simulink library "SIXOSEM_T_STAGE_MASTER"  (Simulink 8.0)
settings: Solver=ode45  StartTime=0.0  StopTime=10.0  RelTol=1e-3
libraries: cdsEpicsOut x51, cdsFilt x31, cdsTP x24, cdsFiltCtrl x9, cdsEpicsIn x9, cdsMuxMatrix x5, cdsEpicsBinIn x2, SIXOSEM_T_COILOUTF_MASTER x1, cdsFunctionCall x1, SIXOSEM_T_WD_AC_MASTER x1
(part 1 of 5)
settings Model: Creator=controls  LastModifiedBy=stuart.aston

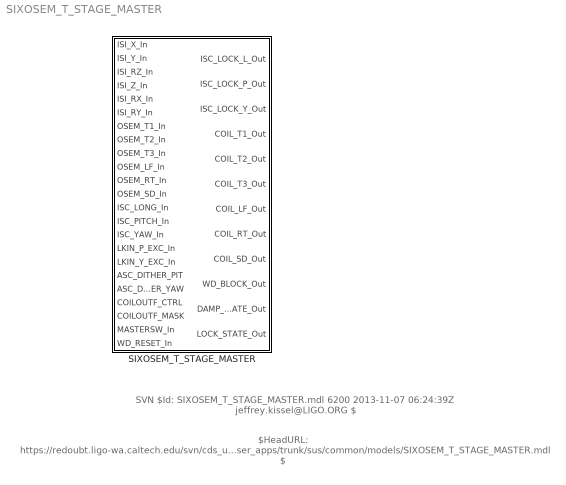
== system SIXOSEM_T_STAGE_MASTER ==
  note: $HeadURL: https://redoubt.ligo-wa.caltech.edu/svn/cds_user_apps/trunk/sus/common/models/SIXOSEM_T_STAGE_MASTER.mdl $
  note: SVN $Id: SIXOSEM_T_STAGE_MASTER.mdl 6200 2013-11-07 06:24:39Z jeffrey.kissel@LIGO.ORG $
  SIXOSEM_T_STAGE_MASTER : Subsystem  Description=SIXOSEMSTAGE_FACE_MASTER

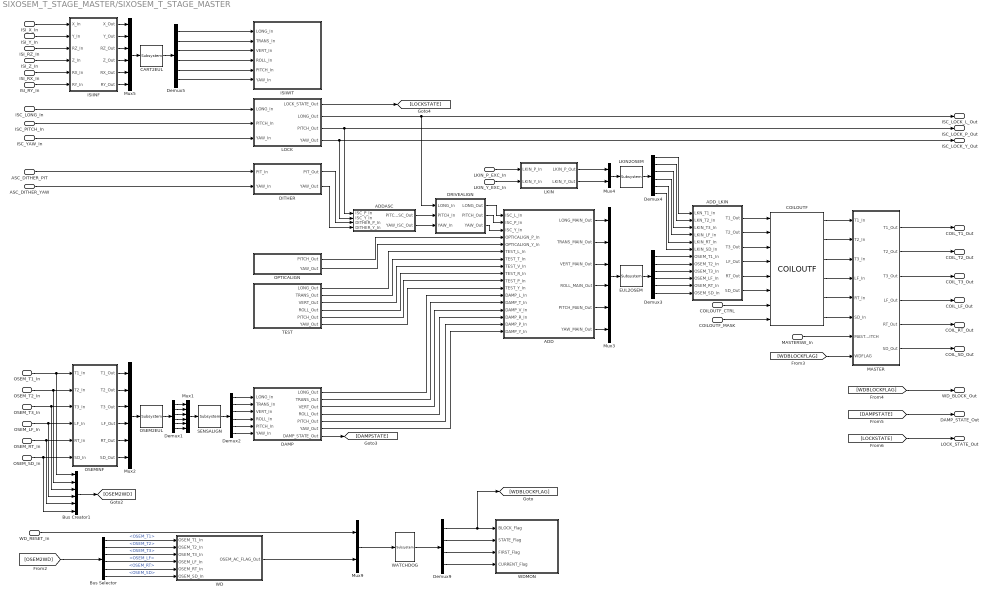
== system SIXOSEM_T_STAGE_MASTER/SIXOSEM_T_STAGE_MASTER ==
  ISI_X_In : Inport
  ISI_Y_In : Inport  Port=2
  ISI_RZ_In : Inport  Port=3
  ISI_Z_In : Inport  Port=4
  ISI_RX_In : Inport  Port=5
  ISI_RY_In : Inport  Port=6
  OSEM_T1_In : Inport  Port=7
  OSEM_T2_In : Inport  Port=8
  OSEM_T3_In : Inport  Port=9
  OSEM_LF_In : Inport  Port=10
  OSEM_RT_In : Inport  Port=11
  OSEM_SD_In : Inport  Port=12
  ISC_LONG_In : Inport  Port=13
  ISC_PITCH_In : Inport  Port=14
  ISC_YAW_In : Inport  Port=15
  LKIN_P_EXC_In : Inport  Port=16
  LKIN_Y_EXC_In : Inport  Port=17
  ASC_DITHER_PIT : Inport  Port=18
  ASC_DITHER_YAW : Inport  Port=19
  COILOUTF_CTRL : Inport  Port=20
  COILOUTF_MASK : Inport  Port=21
  MASTERSW_In : Inport  Port=22
  WD_RESET_In : Inport  Port=23
  ADD : Subsystem
  ADDASC : Subsystem
  ADD_LKIN : Subsystem
  Bus Creator1 : BusCreator  Inputs='OSEM_T1','OSEM_T2','OSEM_T3','OSEM_LF','OSEM_RT','OSEM_SD'
  Bus Selector : BusSelector  OutputSignals=OSEM_T1,OSEM_T2,OSEM_T3,OSEM_LF,OSEM_RT,OSEM_SD
  CART2EUL : cdsMuxMatrix/Subsystem  Tag=cdsMuxMatrix  Description=Any size matrix. Inputs and outputs must be connected using Mux and Demux parts.
      settings: AttributesFormatString=%<Tag>
  COILOUTF : SIXOSEM_T_COILOUTF_MASTER/COILOUTF
  DAMP : Subsystem
  DITHER : Subsystem
  DRIVEALIGN : Subsystem
  Demux{1..5} (5 alike) : Demux  Outputs=6
  Demux9 : Demux
  EUL2OSEM : cdsMuxMatrix/Subsystem  Tag=cdsMuxMatrix  Description=Any size matrix. Inputs and outputs must be connected using Mux and Demux parts.
      settings: AttributesFormatString=%<Tag>
  ISIINF : Subsystem
  ISIWIT : Subsystem
  LKIN : Subsystem
  LKIN2OSEM : cdsMuxMatrix/Subsystem  Tag=cdsMuxMatrix  Description=Any size matrix. Inputs and outputs must be connected using Mux and Demux parts.
      settings: AttributesFormatString=%<Tag>
  LOCK : Subsystem
  MASTER : Subsystem
  Mux{1..3,5} (4 alike) : Mux  Inputs=6
  Mux4 : Mux  Inputs=2
  Mux9 : Mux  Inputs=2
  OPTICALIGN : Subsystem
  OSEM2EUL : cdsMuxMatrix/Subsystem  Tag=cdsMuxMatrix  Description=Any size matrix. Inputs and outputs must be connected using Mux and Demux parts.
      settings: AttributesFormatString=%<Tag>
  OSEMINF : Subsystem
  SENSALIGN : cdsMuxMatrix/Subsystem  Tag=cdsMuxMatrix  Description=Any size matrix. Inputs and outputs must be connected using Mux and Demux parts.
      settings: AttributesFormatString=%<Tag>
  TEST : Subsystem
  WATCHDOG : cdsFunctionCall/Subsystem  Tag=cdsFunctionCall  Description=inline OSEMWATCHDOG $SUS_SRC/WATCHDOG.c
      settings: AttributesFormatString=%<Tag>\n%<Description>
  WD : Subsystem
  WDMON : Subsystem
  ISC_LOCK_L_Out : Outport
  ISC_LOCK_P_Out : Outport  Port=2
  ISC_LOCK_Y_Out : Outport  Port=3
  COIL_T1_Out : Outport  Port=4
  COIL_T2_Out : Outport  Port=5
  COIL_T3_Out : Outport  Port=6
  COIL_LF_Out : Outport  Port=7
  COIL_RT_Out : Outport  Port=8
  COIL_SD_Out : Outport  Port=9
  WD_BLOCK_Out : Outport  Port=10
  DAMP_STATE_Out : Outport  Port=11
  LOCK_STATE_Out : Outport  Port=12
  wires:
  WATCHDOG/1 -> Demux9/1
  Mux9/1 -> WATCHDOG/1
  COILOUTF/6 -> MASTER/6(SD_In)
  COILOUTF/5 -> MASTER/5(RT_In)
  COILOUTF/4 -> MASTER/4(LF_In)
  COILOUTF/3 -> MASTER/3(T3_In)
  COILOUTF/2 -> MASTER/2(T2_In)
  COILOUTF/1 -> MASTER/1(T1_In)
  Demux9/4 -> WDMON/4(CURRENT_Flag)
  Demux9/3 -> WDMON/3(FIRST_Flag)
  Demux9/2 -> WDMON/2(STATE_Flag)
  Demux9/1 -> [WDBLOCKFLAG], WDMON/1(BLOCK_Flag)
  EUL2OSEM/1 -> Demux3/1
  Mux3/1 -> EUL2OSEM/1
  MASTER/6(SD_Out) -> COIL_SD_Out/1
  MASTER/5(RT_Out) -> COIL_RT_Out/1
  MASTER/4(LF_Out) -> COIL_LF_Out/1
  MASTER/3(T3_Out) -> COIL_T3_Out/1
  MASTER/2(T2_Out) -> COIL_T2_Out/1
  MASTER/1(T1_Out) -> COIL_T1_Out/1
  SENSALIGN/1 -> Demux2/1
  Mux1/1 -> SENSALIGN/1
  Demux1/6 -> Mux1/6
  Demux1/5 -> Mux1/5
  Demux1/4 -> Mux1/4
  Demux1/3 -> Mux1/3
  Demux1/2 -> Mux1/2
  Demux1/1 -> Mux1/1
  OSEM2EUL/1 -> Demux1/1
  Bus Selector/6 -> WD/6(OSEM_SD_In)  "<OSEM_SD>"
  Bus Selector/5 -> WD/5(OSEM_RT_In)  "<OSEM_RT>"
  Bus Selector/4 -> WD/4(OSEM_LF_In)  "<OSEM_LF>"
  Bus Selector/3 -> WD/3(OSEM_T3_In)  "<OSEM_T3>"
  Bus Selector/2 -> WD/2(OSEM_T2_In)  "<OSEM_T2>"
  Bus Selector/1 -> WD/1(OSEM_T1_In)  "<OSEM_T1>"
  [OSEM2WD] -> Bus Selector/1
  Bus Creator1/1 -> [OSEM2WD]
  ISC_YAW_In/1 -> LOCK/3(YAW_In)
  ISC_PITCH_In/1 -> LOCK/2(PITCH_In)
  ISC_LONG_In/1 -> LOCK/1(LONG_In)
  Mux2/1 -> OSEM2EUL/1
  OSEM_SD_In/1 -> Bus Creator1/6, OSEMINF/6(SD_In)
  OSEM_RT_In/1 -> Bus Creator1/5, OSEMINF/5(RT_In)
  OSEM_LF_In/1 -> Bus Creator1/4, OSEMINF/4(LF_In)
  OSEM_T3_In/1 -> Bus Creator1/3, OSEMINF/3(T3_In)
  OSEM_T2_In/1 -> Bus Creator1/2, OSEMINF/2(T2_In)
  OSEM_T1_In/1 -> Bus Creator1/1, OSEMINF/1(T1_In)
  OSEMINF/1(T1_Out) -> Mux2/1
  OSEMINF/2(T2_Out) -> Mux2/2
  OSEMINF/3(T3_Out) -> Mux2/3
  OSEMINF/4(LF_Out) -> Mux2/4
  OSEMINF/5(RT_Out) -> Mux2/5
  OSEMINF/6(SD_Out) -> Mux2/6
  ISI_X_In/1 -> ISIINF/1(X_In)
  ISI_Y_In/1 -> ISIINF/2(Y_In)
  ISI_RZ_In/1 -> ISIINF/3(RZ_In)
  ISI_Z_In/1 -> ISIINF/4(Z_In)
  ISI_RX_In/1 -> ISIINF/5(RX_In)
  ISI_RY_In/1 -> ISIINF/6(RY_In)
  ISIINF/1(X_Out) -> Mux5/1
  ISIINF/2(Y_Out) -> Mux5/2
  ISIINF/3(RZ_Out) -> Mux5/3
  ISIINF/4(Z_Out) -> Mux5/4
  ISIINF/5(RX_Out) -> Mux5/5
  ISIINF/6(RY_Out) -> Mux5/6
  Mux5/1 -> CART2EUL/1
  CART2EUL/1 -> Demux5/1
  Demux5/1 -> ISIWIT/1(LONG_In)
  Demux5/2 -> ISIWIT/2(TRANS_In)
  Demux5/3 -> ISIWIT/3(VERT_In)
  Demux5/4 -> ISIWIT/4(ROLL_In)
  Demux5/5 -> ISIWIT/5(PITCH_In)
  Demux5/6 -> ISIWIT/6(YAW_In)
  [WDBLOCKFLAG] -> MASTER/8(WDFLAG)
  Demux2/1 -> DAMP/1(LONG_In)
  Demux2/2 -> DAMP/2(TRANS_In)
  Demux2/3 -> DAMP/3(VERT_In)
  Demux2/4 -> DAMP/4(ROLL_In)
  Demux2/5 -> DAMP/5(PITCH_In)
  Demux2/6 -> DAMP/6(YAW_In)
  [WDBLOCKFLAG] -> WD_BLOCK_Out/1
  DAMP/7(DAMP_STATE_Out) -> [DAMPSTATE]
  [DAMPSTATE] -> DAMP_STATE_Out/1
  ADD/1(LONG_MAIN_Out) -> Mux3/1
  ADD/2(TRANS_MAIN_Out) -> Mux3/2
  ADD/3(VERT_MAIN_Out) -> Mux3/3
  ADD/4(ROLL_MAIN_Out) -> Mux3/4
  ADD/5(PITCH_MAIN_Out) -> Mux3/5
  ADD/6(YAW_MAIN_Out) -> Mux3/6
  LOCK/1(LOCK_STATE_Out) -> [LOCKSTATE]
  [LOCKSTATE] -> LOCK_STATE_Out/1
  LKIN/1(LKIN_P_Out) -> Mux4/1
  LKIN2OSEM/1 -> Demux4/1
  Mux4/1 -> LKIN2OSEM/1
  ADD_LKIN/1(T1_Out) -> COILOUTF/1
  ADD_LKIN/2(T2_Out) -> COILOUTF/2
  ADD_LKIN/3(T3_Out) -> COILOUTF/3
  ADD_LKIN/4(LF_Out) -> COILOUTF/4
  ADD_LKIN/5(RT_Out) -> COILOUTF/5
  ADD_LKIN/6(SD_Out) -> COILOUTF/6
  Demux4/1 -> ADD_LKIN/1(LKN_T1_In)
  Demux4/2 -> ADD_LKIN/2(LKN_T2_In)
  Demux4/3 -> ADD_LKIN/3(LKIN_T3_In)
  Demux4/4 -> ADD_LKIN/4(LKIN_LF_In)
  Demux4/5 -> ADD_LKIN/5(LKIN_RT_In)
  Demux4/6 -> ADD_LKIN/6(LKIN_SD_In)
  Demux3/1 -> ADD_LKIN/7(OSEM_T1_In)
  Demux3/2 -> ADD_LKIN/8(OSEM_T2_In)
  Demux3/3 -> ADD_LKIN/9(OSEM_T3_In)
  Demux3/4 -> ADD_LKIN/10(OSEM_LF_In)
  Demux3/5 -> ADD_LKIN/11(OSEM_RT_In)
  Demux3/6 -> ADD_LKIN/12(OSEM_SD_In)
  MASTERSW_In/1 -> MASTER/7(MASTERSWITCH)
  COILOUTF_MASK/1 -> COILOUTF/8
  COILOUTF_CTRL/1 -> COILOUTF/7
  LKIN/2(LKIN_Y_Out) -> Mux4/2
  LKIN_P_EXC_In/1 -> LKIN/1(LKIN_P_In)
  LKIN_Y_EXC_In/1 -> LKIN/2(LKIN_Y_In)
  DRIVEALIGN/1(LONG_Out) -> ADD/1(ISC_L_In)
  DRIVEALIGN/2(PITCH_Out) -> ADD/2(ISC_P_In)
  DRIVEALIGN/3(YAW_Out) -> ADD/3(ISC_Y_In)
  LOCK/2(LONG_Out) -> DRIVEALIGN/1(LONG_In), ISC_LOCK_L_Out/1
  LOCK/3(PITCH_Out) -> ISC_LOCK_P_Out/1, ADDASC/1(ISC_P_In)
  LOCK/4(YAW_Out) -> ADDASC/2(ISC_Y_In), ISC_LOCK_Y_Out/1
  WD/1(OSEM_AC_FLAG_Out) -> Mux9/2
  WD_RESET_In/1 -> Mux9/1
  ASC_DITHER_PIT/1 -> DITHER/1(PIT_In)
  ASC_DITHER_YAW/1 -> DITHER/2(YAW_In)
  ADDASC/1(PITCH_ISC_Out) -> DRIVEALIGN/2(PITCH_In)
  ADDASC/2(YAW_ISC_Out) -> DRIVEALIGN/3(YAW_In)
  DITHER/1(PIT_Out) -> ADDASC/3(DITHER_P_In)
  DITHER/2(YAW_Out) -> ADDASC/4(DITHER_Y_In)
  OPTICALIGN/1(PITCH_Out) -> ADD/4(OPTICALIGN_P_In)
  OPTICALIGN/2(YAW_Out) -> ADD/5(OPTICALIGN_Y_In)
  TEST/1(LONG_Out) -> ADD/6(TEST_L_In)
  TEST/2(TRANS_Out) -> ADD/7(TEST_T_In)
  TEST/3(VERT_Out) -> ADD/8(TEST_V_In)
  TEST/4(ROLL_Out) -> ADD/9(TEST_R_In)
  TEST/5(PITCH_Out) -> ADD/10(TEST_P_In)
  TEST/6(YAW_Out) -> ADD/11(TEST_Y_In)
  DAMP/1(LONG_Out) -> ADD/12(DAMP_L_In)
  DAMP/2(TRANS_Out) -> ADD/13(DAMP_T_In)
  DAMP/3(VERT_Out) -> ADD/14(DAMP_V_In)
  DAMP/4(ROLL_Out) -> ADD/15(DAMP_R_In)
  DAMP/5(PITCH_Out) -> ADD/16(DAMP_P_In)
  DAMP/6(YAW_Out) -> ADD/17(DAMP_Y_In)

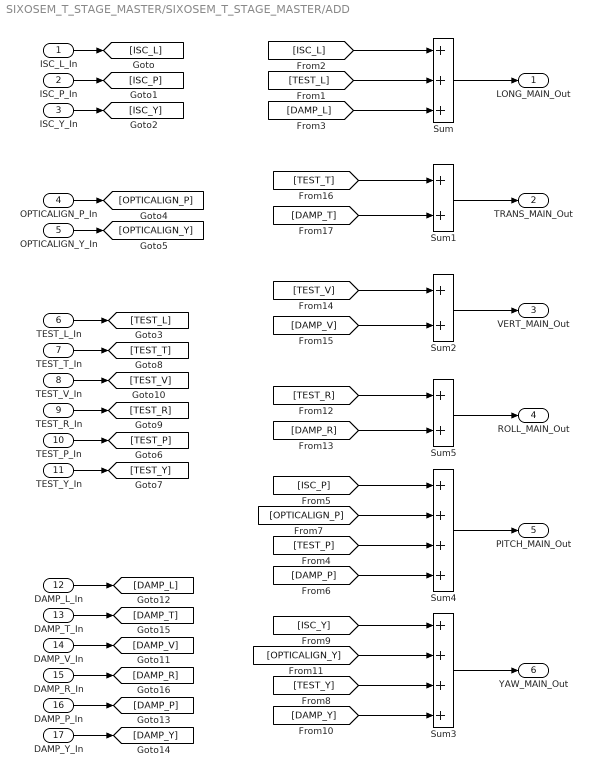
== system SIXOSEM_T_STAGE_MASTER/SIXOSEM_T_STAGE_MASTER/ADD ==
  ISC_L_In : Inport
  ISC_P_In : Inport  Port=2
  ISC_Y_In : Inport  Port=3
  OPTICALIGN_P_In : Inport  Port=4
  OPTICALIGN_Y_In : Inport  Port=5
  TEST_L_In : Inport  Port=6
  TEST_T_In : Inport  Port=7
  TEST_V_In : Inport  Port=8
  TEST_R_In : Inport  Port=9
  TEST_P_In : Inport  Port=10
  TEST_Y_In : Inport  Port=11
  DAMP_L_In : Inport  Port=12
  DAMP_T_In : Inport  Port=13
  DAMP_V_In : Inport  Port=14
  DAMP_R_In : Inport  Port=15
  DAMP_P_In : Inport  Port=16
  DAMP_Y_In : Inport  Port=17
  Sum : Sum  Inputs=+++
  Sum1 : Sum
  Sum2 : Sum
  Sum3 : Sum  Inputs=++++
  Sum4 : Sum  Inputs=++++
  Sum5 : Sum
  LONG_MAIN_Out : Outport
  TRANS_MAIN_Out : Outport  Port=2
  VERT_MAIN_Out : Outport  Port=3
  ROLL_MAIN_Out : Outport  Port=4
  PITCH_MAIN_Out : Outport  Port=5
  YAW_MAIN_Out : Outport  Port=6
  wires:
  Sum4/1 -> PITCH_MAIN_Out/1
  Sum3/1 -> YAW_MAIN_Out/1
  Sum/1 -> LONG_MAIN_Out/1
  [ISC_L] -> Sum/1
  [TEST_L] -> Sum/2
  [DAMP_L] -> Sum/3
  Sum5/1 -> ROLL_MAIN_Out/1
  Sum2/1 -> VERT_MAIN_Out/1
  Sum1/1 -> TRANS_MAIN_Out/1
  OPTICALIGN_P_In/1 -> [OPTICALIGN_P]
  OPTICALIGN_Y_In/1 -> [OPTICALIGN_Y]
  ISC_L_In/1 -> [ISC_L]
  ISC_P_In/1 -> [ISC_P]
  ISC_Y_In/1 -> [ISC_Y]
  TEST_L_In/1 -> [TEST_L]
  TEST_T_In/1 -> [TEST_T]
  TEST_V_In/1 -> [TEST_V]
  TEST_R_In/1 -> [TEST_R]
  TEST_P_In/1 -> [TEST_P]
  TEST_Y_In/1 -> [TEST_Y]
  DAMP_L_In/1 -> [DAMP_L]
  DAMP_T_In/1 -> [DAMP_T]
  DAMP_V_In/1 -> [DAMP_V]
  DAMP_R_In/1 -> [DAMP_R]
  DAMP_P_In/1 -> [DAMP_P]
  DAMP_Y_In/1 -> [DAMP_Y]
  [ISC_P] -> Sum4/1
  [OPTICALIGN_P] -> Sum4/2
  [TEST_P] -> Sum4/3
  [DAMP_P] -> Sum4/4
  [ISC_Y] -> Sum3/1
  [OPTICALIGN_Y] -> Sum3/2
  [TEST_Y] -> Sum3/3
  [DAMP_Y] -> Sum3/4
  [TEST_R] -> Sum5/1
  [DAMP_R] -> Sum5/2
  [TEST_T] -> Sum1/1
  [DAMP_T] -> Sum1/2
  [TEST_V] -> Sum2/1
  [DAMP_V] -> Sum2/2

== system SIXOSEM_T_STAGE_MASTER/SIXOSEM_T_STAGE_MASTER/ADDASC ==
  ISC_P_In : Inport
  ISC_Y_In : Inport  Port=2
  DITHER_P_In : Inport  Port=3
  DITHER_Y_In : Inport  Port=4
  Sum1 : Sum
  Sum2 : Sum
  PITCH_ISC_Out : Outport
  YAW_ISC_Out : Outport  Port=2
  wires:
  [DITHER_Y] -> Sum2/2
  [ISC_Y] -> Sum2/1
  [DITHER_P] -> Sum1/2
  [ISC_P] -> Sum1/1
  ISC_Y_In/1 -> [ISC_Y]
  ISC_P_In/1 -> [ISC_P]
  DITHER_Y_In/1 -> [DITHER_Y]
  DITHER_P_In/1 -> [DITHER_P]
  Sum1/1 -> PITCH_ISC_Out/1
  Sum2/1 -> YAW_ISC_Out/1

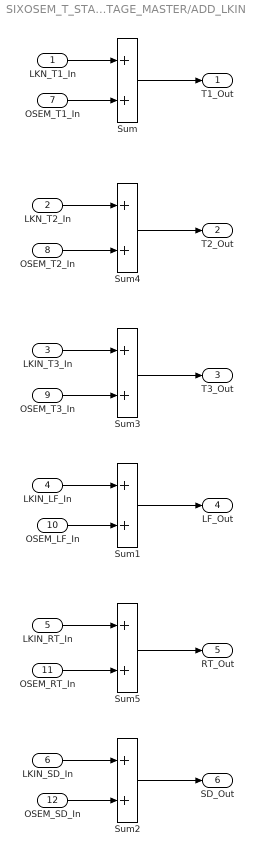
== system SIXOSEM_T_STAGE_MASTER/SIXOSEM_T_STAGE_MASTER/ADD_LKIN ==
  LKN_T1_In : Inport
  LKN_T2_In : Inport  Port=2
  LKIN_T3_In : Inport  Port=3
  LKIN_LF_In : Inport  Port=4
  LKIN_RT_In : Inport  Port=5
  LKIN_SD_In : Inport  Port=6
  OSEM_T1_In : Inport  Port=7
  OSEM_T2_In : Inport  Port=8
  OSEM_T3_In : Inport  Port=9
  OSEM_LF_In : Inport  Port=10
  OSEM_RT_In : Inport  Port=11
  OSEM_SD_In : Inport  Port=12
  Sum{,1..5} (6 alike) : Sum
  T1_Out : Outport
  T2_Out : Outport  Port=2
  T3_Out : Outport  Port=3
  LF_Out : Outport  Port=4
  RT_Out : Outport  Port=5
  SD_Out : Outport  Port=6
  wires:
  OSEM_LF_In/1 -> Sum1/2
  Sum1/1 -> LF_Out/1
  OSEM_T2_In/1 -> Sum4/2
  OSEM_T3_In/1 -> Sum3/2
  Sum4/1 -> T2_Out/1
  Sum3/1 -> T3_Out/1
  OSEM_T1_In/1 -> Sum/2
  LKN_T1_In/1 -> Sum/1
  Sum/1 -> T1_Out/1
  LKN_T2_In/1 -> Sum4/1
  LKIN_T3_In/1 -> Sum3/1
  LKIN_LF_In/1 -> Sum1/1
  OSEM_SD_In/1 -> Sum2/2
  Sum2/1 -> SD_Out/1
  OSEM_RT_In/1 -> Sum5/2
  Sum5/1 -> RT_Out/1
  LKIN_RT_In/1 -> Sum5/1
  LKIN_SD_In/1 -> Sum2/1
